simulink model "Q1_UAV"  (R2022a)
settings: Solver=VariableStepAuto  StartTime=0.0  StopTime=10  RelTol=1e-3
settings Model: Creator=Eshmith  LastModifiedBy=Eshmith

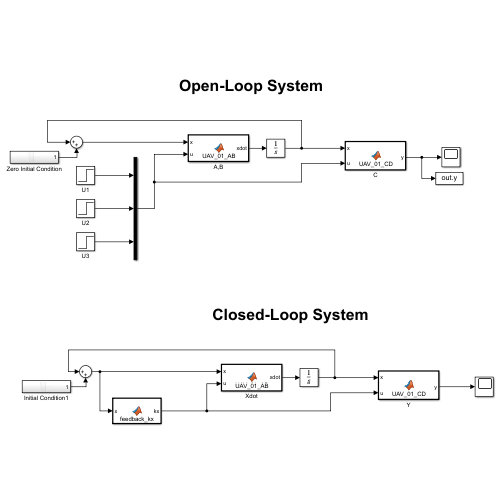
[thumbnail: Simulink's stored preview of the top-level diagram]
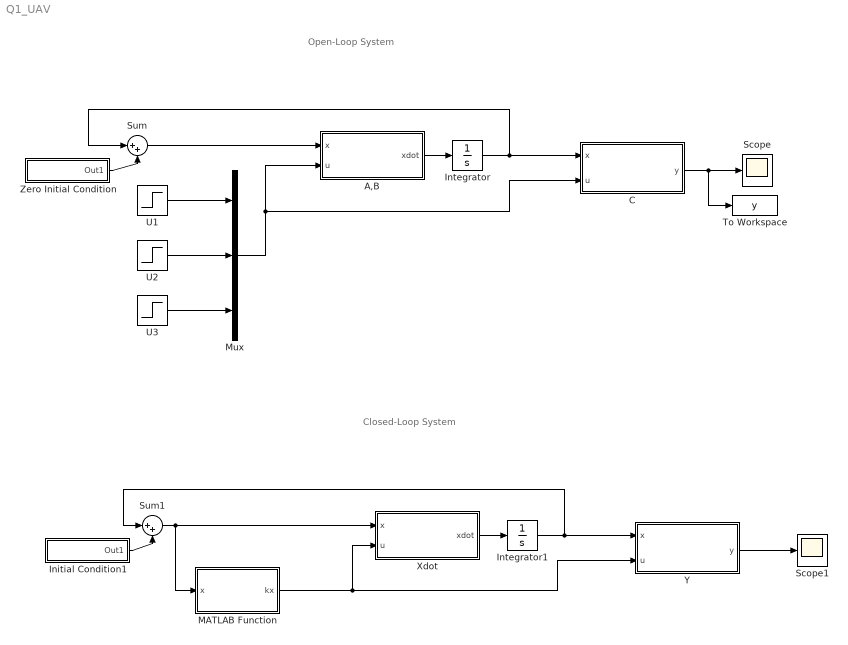
== system Q1_UAV ==
  note: Open-Loop System
  note: Closed-Loop System
  A,B : MATLAB Function  TreatAsAtomicUnit=on
  C : MATLAB Function  TreatAsAtomicUnit=on
  Initial Condition1 : Subsystem
  Integrator : Integrator
  Integrator1 : Integrator
  MATLAB Function : MATLAB Function  TreatAsAtomicUnit=on
  Mux : Mux  Inputs=3
  Scope : Scope
  Scope1 : Scope
  Sum : Sum  Inputs=|++
  Sum1 : Sum  Inputs=|++
  To Workspace : ToWorkspace  VariableName=y  SaveFormat=Timeseries  SampleTime=-1
  U1 : Step  Time=0  SampleTime=0
  U2 : Step  Time=0  After=0  SampleTime=0
  U3 : Step  After=0  SampleTime=0
  Xdot : MATLAB Function  TreatAsAtomicUnit=on
  Y : MATLAB Function  TreatAsAtomicUnit=on
  Zero Initial Condition : Subsystem
  wires:
  A,B/1(xdot) -> Integrator/1
  U1/1 -> Mux/1
  Mux/1 -> A,B/2(u), C/2(u)
  Integrator/1 -> Sum/1, C/1(x)
  C/1(y) -> To Workspace/1, Scope/1
  Sum/1 -> A,B/1(x)
  Zero Initial Condition/1(Out1) -> Sum/2
  U2/1 -> Mux/2
  U3/1 -> Mux/3
  Sum1/1 -> MATLAB Function/1(x), Xdot/1(x)
  Integrator1/1 -> Sum1/1, Y/1(x)
  Y/1(y) -> Scope1/1
  Initial Condition1/1(Out1) -> Sum1/2
  Xdot/1(xdot) -> Integrator1/1
  MATLAB Function/1(kx) -> Y/2(u), Xdot/2(u)

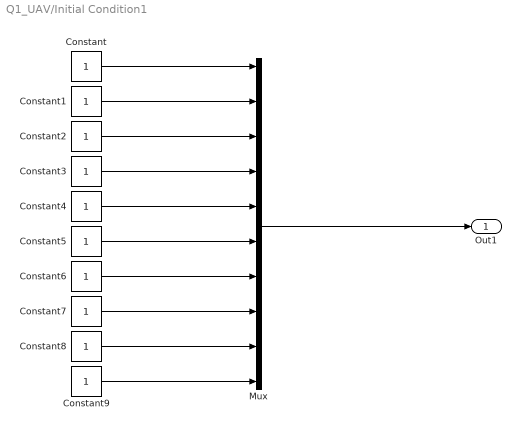
== system Q1_UAV/Initial Condition1 ==
  Constant{,1..9} (10 alike) : Constant
  Mux : Mux  Inputs=10
  Out1 : Outport
  wires:
  Mux/1 -> Out1/1
  Constant5/1 -> Mux/6
  Constant7/1 -> Mux/8
  Constant2/1 -> Mux/3
  Constant9/1 -> Mux/10
  Constant3/1 -> Mux/4
  Constant8/1 -> Mux/9
  Constant1/1 -> Mux/2
  Constant/1 -> Mux/1
  Constant4/1 -> Mux/5
  Constant6/1 -> Mux/7

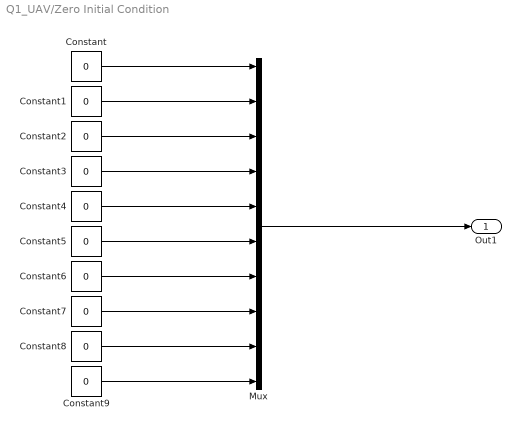
== system Q1_UAV/Zero Initial Condition ==
  Constant{,1..9} (10 alike) : Constant  Value=0
  Mux : Mux  Inputs=10
  Out1 : Outport
  wires:
  Mux/1 -> Out1/1
  Constant5/1 -> Mux/6
  Constant7/1 -> Mux/8
  Constant2/1 -> Mux/3
  Constant9/1 -> Mux/10
  Constant3/1 -> Mux/4
  Constant8/1 -> Mux/9
  Constant1/1 -> Mux/2
  Constant/1 -> Mux/1
  Constant4/1 -> Mux/5
  Constant6/1 -> Mux/7

== matlab function Q1_UAV/A,B ==
  data: x input; u input; xdot output
function xdot = UAV_01_AB(x, u)

A = [-1.9,0,-0.68,0,0,0,0,0,0,0.3065;
      0,-8.9,0,0.1812,-3.944,0,0,0,0,0;
     -0.044,0,-2.82,0,0,0,0,0,0,1.223;
      0,-11.48,0,-0.009451,-0.06638,0,0,0,-9.79,0;
      0,2487,0,-0.02051,-1.034,0,0,0,-0.4497,0;
      0,0,0,0.04589,-0.9989,0.0,0,-0.00,2503,0;
      1,0,0.04593,0,0,0,0,0,0,0;
      0,0,1.001,0,0,0,0,0,0,0;
      0,1,0,0,0,0,0,0,0,0;
      11.48,0,-2484,0,0,0,9.79,0,0,-1.054;
    ];

B = [0,100,100;
     1100,0,0;
     0,2.10,100;
     10.0,0,0;
     10.0,0,0;
     0,0,0;
     0,0,0;
     0,0,00;
     0,0,0;
     0,-0.001,-10.2;
    ];

K = ones(3, 10);

xdot = A*x + B*u;

end

== matlab function Q1_UAV/Xdot ==
  data: x input; u input; xdot output
function xdot = UAV_01_AB(x, u)

A = [-1.9,0,-0.68,0,0,0,0,0,0,0.3065;
      0,-8.9,0,0.1812,-3.944,0,0,0,0,0;
     -0.044,0,-2.82,0,0,0,0,0,0,1.223;
      0,-11.48,0,-0.009451,-0.06638,0,0,0,-9.79,0;
      0,2487,0,-0.02051,-1.034,0,0,0,-0.4497,0;
      0,0,0,0.04589,-0.9989,0.0,0,-0.00,2503,0;
      1,0,0.04593,0,0,0,0,0,0,0;
      0,0,1.001,0,0,0,0,0,0,0;
      0,1,0,0,0,0,0,0,0,0;
      11.48,0,-2484,0,0,0,9.79,0,0,-1.054;
    ];

B = [0,100,100;
     1100,0,0;
     0,2.10,100;
     10.0,0,0;
     10.0,0,0;
     0,0,0;
     0,0,0;
     0,0,00;
     0,0,0;
     0,-0.001,-10.2;
    ];

K = ones(3, 10);

xdot = A*x + B*u;

end

== matlab function Q1_UAV/Y ==
  data: x input; u input; y output
function y = UAV_01_CD(x, u)

y1 = [0 0 0 0 0 0 1 0 0 0];
C = [y1; circshift(y1,1); circshift(y1,2)];

D = zeros(3,3);

K = ones(3, 10);

y = C*x + D*u;

end

== matlab function Q1_UAV/MATLAB Function ==
  data: x input; kx output
function kx = feedback_kx(x)

K = ones(3,10);

kx = -K*x;

end

== matlab function Q1_UAV/C ==
  data: x input; u input; y output
function y = UAV_01_CD(x, u)

y1 = [0 0 0 0 0 0 1 0 0 0];
C = [y1; circshift(y1,1); circshift(y1,2)];

D = zeros(3,3);

K = ones(3, 10);

y = C*x + D*u;

end
